simulink model "TST_PthSet_OvrRunCoord"  (R2016b)
settings: Solver=FixedStepDiscrete  StartTime=0.0  StopTime=simTime  FixedStep=sampleTime  RelTol=1e-3
values from neighbouring files (symbols this model uses):
  testCase = 1    [initTST_PthSet_OvrRunCoord_001.m]
libraries: simulink x3, UnitTest_Lib x1
settings Model: Creator=zhengjinyan  LastModifiedBy=zhengjinyan
settings DebuggingCC: SignalRangeChecking=error

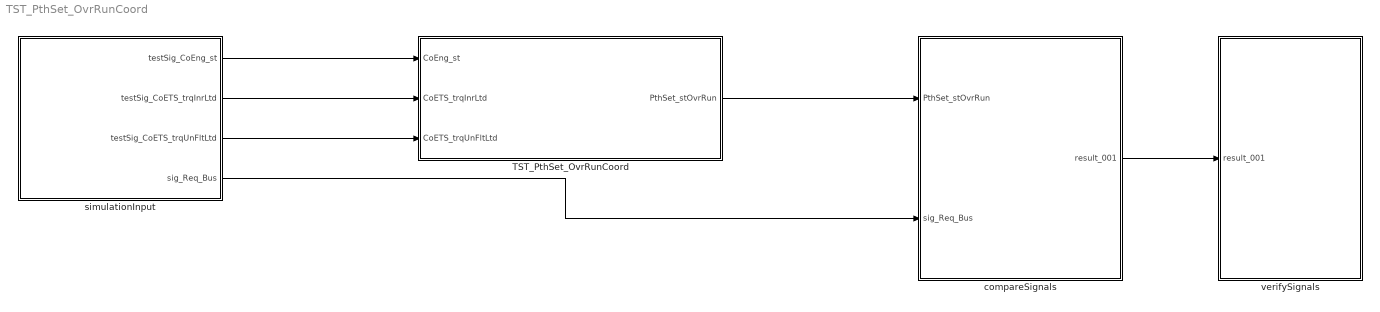
== system TST_PthSet_OvrRunCoord ==
  TST_PthSet_OvrRunCoord : Subsystem
  compareSignals : Subsystem
  simulationInput : Subsystem
  verifySignals : Subsystem
  wires:
  simulationInput/1(testSig_CoEng_st) -> TST_PthSet_OvrRunCoord/1(CoEng_st)
  simulationInput/2(testSig_CoETS_trqInrLtd) -> TST_PthSet_OvrRunCoord/2(CoETS_trqInrLtd)
  simulationInput/3(testSig_CoETS_trqUnFltLtd) -> TST_PthSet_OvrRunCoord/3(CoETS_trqUnFltLtd)
  TST_PthSet_OvrRunCoord/1(PthSet_stOvrRun) -> compareSignals/1(PthSet_stOvrRun)
  simulationInput/4(sig_Req_Bus) -> compareSignals/2(sig_Req_Bus)
  compareSignals/1(result_001) -> verifySignals/1(result_001)

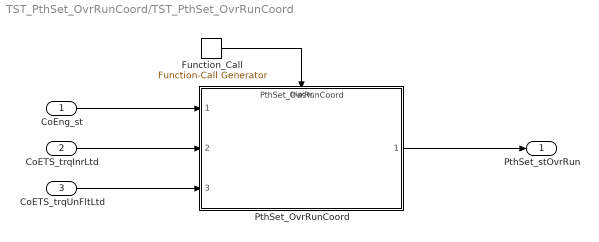
== system TST_PthSet_OvrRunCoord/TST_PthSet_OvrRunCoord ==
  CoEng_st : Inport
  CoETS_trqInrLtd : Inport  Port=2
  CoETS_trqUnFltLtd : Inport  Port=3
  Function_Call : simulink/Ports & Subsystems/Function-Call Generator  sample_time=sampleTime  numberOfIterations=1
  PthSet_OvrRunCoord : ModelReference  ModelNameDialog=PthSet_OvrRunCoord  SimulationMode=Normal  ModelReferenceVersion=1.2  TriggerPortName=function  TriggerPortTriggerType=function-call  TriggerPortStatesWhenEnabling=held
  PthSet_stOvrRun : Outport
  wires:
  Function_Call/1 -> PthSet_OvrRunCoord/Trigger
  CoEng_st/1 -> PthSet_OvrRunCoord/1
  CoETS_trqInrLtd/1 -> PthSet_OvrRunCoord/2
  CoETS_trqUnFltLtd/1 -> PthSet_OvrRunCoord/3
  PthSet_OvrRunCoord/1 -> PthSet_stOvrRun/1

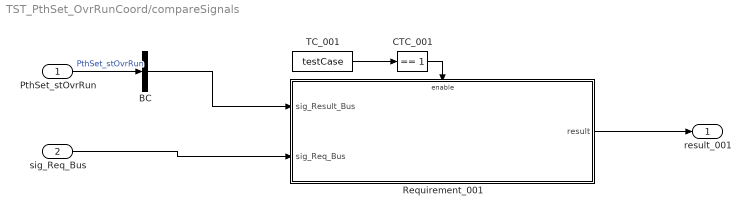
== system TST_PthSet_OvrRunCoord/compareSignals ==
  PthSet_stOvrRun : Inport
  sig_Req_Bus : Inport  Port=2
  BC : BusCreator  Inputs=1
  CTC_001 : simulink/Logic and Bit Operations/Compare To Constant  relop===  const=1  OutDataTypeStr=boolean
  Requirement_001 : Subsystem
  TC_001 : Constant  Value=testCase
  result_001 : Outport
  wires:
  PthSet_stOvrRun/1 -> BC/1  "PthSet_stOvrRun"
  TC_001/1 -> CTC_001/1
  CTC_001/1 -> Requirement_001/Enable
  sig_Req_Bus/1 -> Requirement_001/2(sig_Req_Bus)
  BC/1 -> Requirement_001/1(sig_Result_Bus)
  Requirement_001/1(result) -> result_001/1

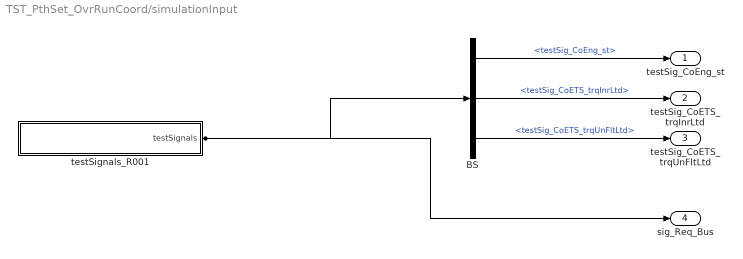
== system TST_PthSet_OvrRunCoord/simulationInput ==
  BS : BusSelector  OutputSignals=testSig_CoEng_st,testSig_CoETS_trqInrLtd,testSig_CoETS_trqUnFltLtd
  testSignals_R001 : Subsystem
  testSig_CoEng_st : Outport
  testSig_CoETS_trqInrLtd : Outport  Port=2
  testSig_CoETS_trqUnFltLtd : Outport  Port=3
  sig_Req_Bus : Outport  Port=4
  wires:
  BS/1 -> testSig_CoEng_st/1  "<testSig_CoEng_st>"
  BS/2 -> testSig_CoETS_trqInrLtd/1  "<testSig_CoETS_trqInrLtd>"
  BS/3 -> testSig_CoETS_trqUnFltLtd/1  "<testSig_CoETS_trqUnFltLtd>"
  testSignals_R001/1(testSignals) -> BS/1, sig_Req_Bus/1

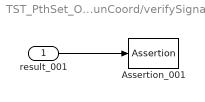
== system TST_PthSet_OvrRunCoord/verifySignals ==
  result_001 : Inport
  Assertion_001 : Assertion  Enabled=off
  wires:
  result_001/1 -> Assertion_001/1

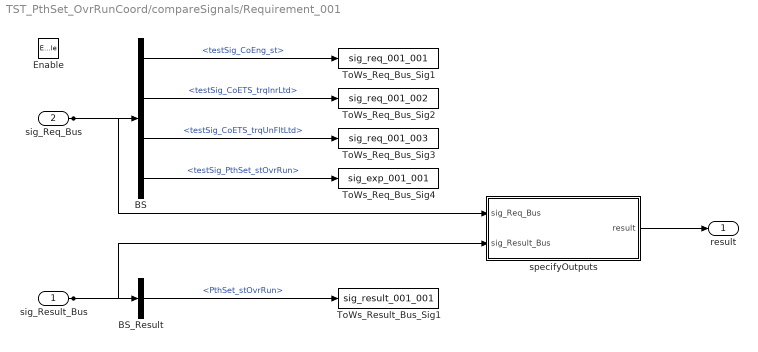
== system TST_PthSet_OvrRunCoord/compareSignals/Requirement_001 ==
  sig_Result_Bus : Inport
  sig_Req_Bus : Inport  Port=2
  Enable : EnablePort
  BS : BusSelector  OutputSignals=testSig_CoEng_st,testSig_CoETS_trqInrLtd,testSig_CoETS_trqUnFltLtd,testSig_PthSet_stOvrRun
  BS_Result : BusSelector  OutputSignals=PthSet_stOvrRun
  ToWs_Req_Bus_Sig1 : ToWorkspace  VariableName=sig_req_001_001  SaveFormat=Structure With Time
  ToWs_Req_Bus_Sig2 : ToWorkspace  VariableName=sig_req_001_002  SaveFormat=Structure With Time
  ToWs_Req_Bus_Sig3 : ToWorkspace  VariableName=sig_req_001_003  SaveFormat=Structure With Time
  ToWs_Req_Bus_Sig4 : ToWorkspace  VariableName=sig_exp_001_001  SaveFormat=Structure With Time
  ToWs_Result_Bus_Sig1 : ToWorkspace  VariableName=sig_result_001_001  SaveFormat=Structure With Time
  specifyOutputs : Subsystem
  result : Outport
  wires:
  sig_Req_Bus/1 -> BS/1, specifyOutputs/1(sig_Req_Bus)
  BS/1 -> ToWs_Req_Bus_Sig1/1  "<testSig_CoEng_st>"
  BS/2 -> ToWs_Req_Bus_Sig2/1  "<testSig_CoETS_trqInrLtd>"
  BS/3 -> ToWs_Req_Bus_Sig3/1  "<testSig_CoETS_trqUnFltLtd>"
  BS/4 -> ToWs_Req_Bus_Sig4/1  "<testSig_PthSet_stOvrRun>"
  sig_Result_Bus/1 -> BS_Result/1, specifyOutputs/2(sig_Result_Bus)
  BS_Result/1 -> ToWs_Result_Bus_Sig1/1  "<PthSet_stOvrRun>"
  specifyOutputs/1(result) -> result/1

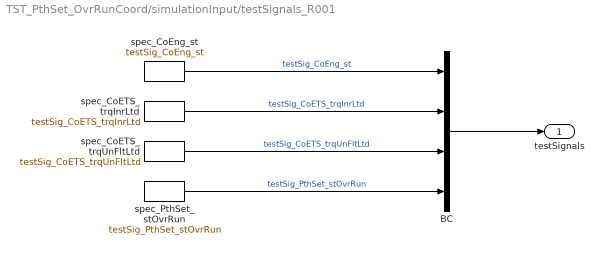
== system TST_PthSet_OvrRunCoord/simulationInput/testSignals_R001 ==
  BC : BusCreator  Inputs=4
  spec_CoETS_trqInrLtd : FromWorkspace  VariableName=testSig_CoETS_trqInrLtd  Interpolate=off  OutputAfterFinalValue=Holding final value
  spec_CoETS_trqUnFltLtd : FromWorkspace  VariableName=testSig_CoETS_trqUnFltLtd  Interpolate=off  OutputAfterFinalValue=Holding final value
  spec_CoEng_st : FromWorkspace  VariableName=testSig_CoEng_st  Interpolate=off  OutputAfterFinalValue=Holding final value
  spec_PthSet_stOvrRun : FromWorkspace  VariableName=testSig_PthSet_stOvrRun  Interpolate=off  OutputAfterFinalValue=Holding final value
  testSignals : Outport
  wires:
  BC/1 -> testSignals/1
  spec_CoEng_st/1 -> BC/1  "testSig_CoEng_st"
  spec_CoETS_trqInrLtd/1 -> BC/2  "testSig_CoETS_trqInrLtd"
  spec_CoETS_trqUnFltLtd/1 -> BC/3  "testSig_CoETS_trqUnFltLtd"
  spec_PthSet_stOvrRun/1 -> BC/4  "testSig_PthSet_stOvrRun"

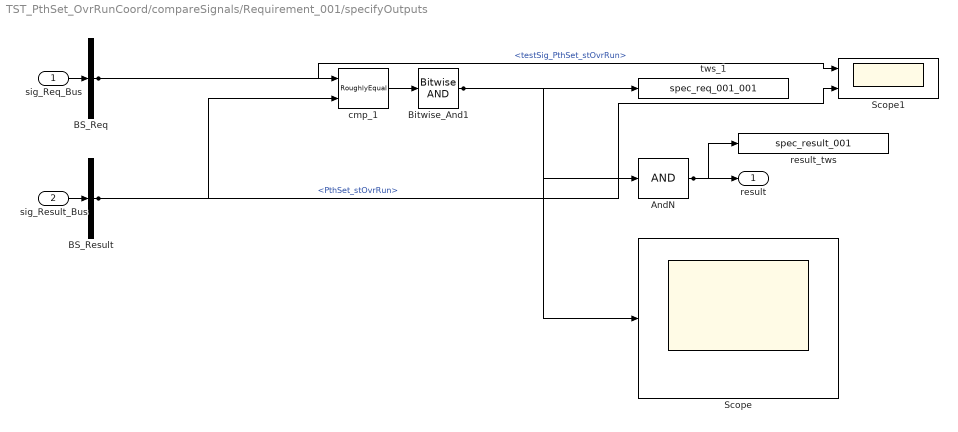
== system TST_PthSet_OvrRunCoord/compareSignals/Requirement_001/specifyOutputs ==
  sig_Req_Bus : Inport
  sig_Result_Bus : Inport  Port=2
  AndN : Logic  Inputs=1
  BS_Req : BusSelector  OutputSignals=testSig_PthSet_stOvrRun
  BS_Result : BusSelector  OutputSignals=PthSet_stOvrRun
  Bitwise_And1 : simulink/Logic and Bit Operations/Bitwise Operator  logicop=AND  UseBitMask=off  BitMask=bin2dec('11011001')  BitMaskRealWorld=Stored Integer
  Scope : Scope
  Scope1 : Scope  NumInputPorts=2
  cmp_1 : UnitTest_Lib/RoughlyEqual  slope=0.1
  result_tws : ToWorkspace  VariableName=spec_result_001
  tws_1 : ToWorkspace  VariableName=spec_req_001_001
  result : Outport
  wires:
  sig_Req_Bus/1 -> BS_Req/1
  sig_Result_Bus/1 -> BS_Result/1
  AndN/1 -> result/1, result_tws/1
  BS_Req/1 -> cmp_1/1, Scope1/1  "<testSig_PthSet_stOvrRun>"
  BS_Result/1 -> cmp_1/2, Scope1/2  "<PthSet_stOvrRun>"
  cmp_1/1 -> Bitwise_And1/1
  Bitwise_And1/1 -> tws_1/1, AndN/1, Scope/1
